simulink model "Lab03IntControleCOMPLETO"  (R2021a)
settings: Solver=ode45  StartTime=0.0  StopTime=150  RelTol=1e-3  EnableMultiTasking=on
settings Model: Creator=13199959938  LastModifiedBy=Usuario
settings SolverCC: AlgebraicLoopSolver=TrustRegion
settings DataIOCC: LimitDataPoints=on  SaveFormat=Array  ReturnWorkspaceOutputs=off
settings OptimizationCC: LifeSpan=inf
settings DebuggingCC: UnderspecifiedInitializationDetection=Classic  MergeDetectMultiDrivingBlocksExec=none  SolverPrmCheckMsg=warning  StateNameClashWarn=warning  SFUnexpectedBacktrackingDiag=warning  SFNoUnconditionalDefaultTransitionDiag=warning  SFExecutionAtInitializationDiag=none  SFMachineParentedDataDiag=warning  ArithmeticOperatorsInVariantConditions=warning
settings HardwareCC: ProdBitPerPointer=32  ProdBitPerSizeT=32  ProdBitPerPtrDiffT=32  ProdLargestAtomicFloat=None  ProdIntDivRoundTo=Undefined  ProdEndianess=Unspecified  ProdWordSize=32  ProdHWDeviceType=32-bit Generic
settings ModelReferenceCC: PropagateSignalLabelsOutOfModel=off
settings SFSimCC: SimUseLocalCustomCode=off  CustomCodeUndefinedFunction=UseInterfaceOnly
settings RTWCC: RTWUseLocalCustomCode=off
settings CodeAppCC: StateflowObjectComments=on
settings GRTTargetCC: TargetLangStandard=C89/C90 (ANSI)
settings ConfigComp: CovMetricSettings=dw  CovSaveCumulativeToWorkspaceVar=on  CovSaveSingleToWorkspaceVar=on  CovExternalEMLEnable=off

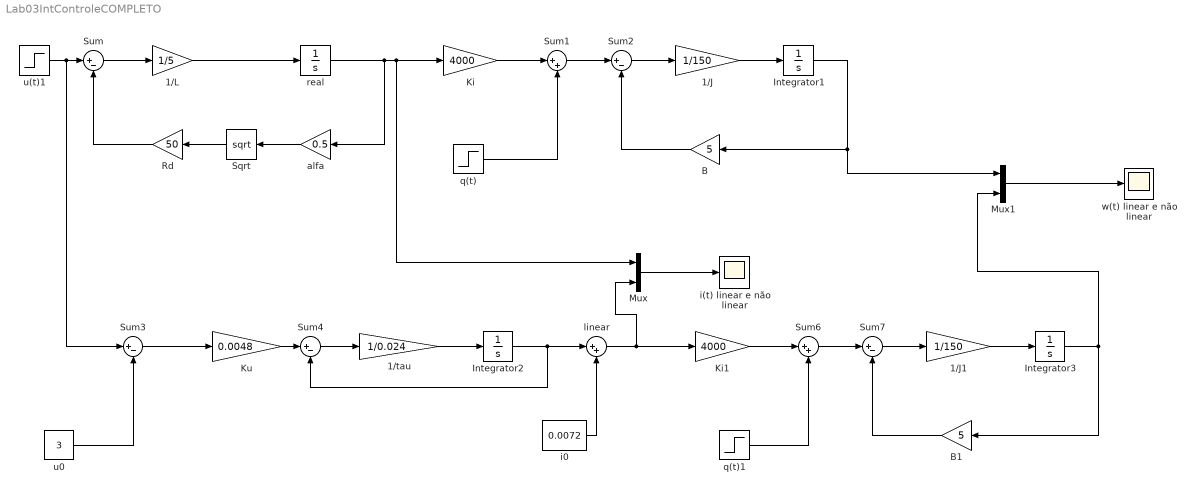
== system Lab03IntControleCOMPLETO ==
  1/J : Gain  Gain=1/150
  1/J1 : Gain  Gain=1/150
  1/L : Gain  Gain=1/5
  1/tau : Gain  Gain=1/0.024
  B : Gain  Gain=5
  B1 : Gain  Gain=5
  Integrator1 : Integrator
  Integrator2 : Integrator
  Integrator3 : Integrator
  Ki : Gain  Gain=4000
  Ki1 : Gain  Gain=4000
  Ku : Gain  Gain=0.0048
  Mux : Mux  Inputs=2
  Mux1 : Mux  Inputs=2
  Rd : Gain  Gain=50
  Sqrt : Sqrt  SaturateOnIntegerOverflow=on
  Sum{,2..4,7} (5 alike) : Sum  Inputs=|+-
  Sum1 : Sum  Inputs=|++
  Sum6 : Sum  Inputs=|++
  alfa : Gain  Gain=0.5
  i(t) linear e não linear : Scope
  i0 : Constant  Value=0.0072
  linear : Sum  Inputs=|++
  q(t) : Step  Time=50  After=0  SampleTime=0
  q(t)1 : Step  Time=50  SampleTime=0
  real : Integrator
  u(t)1 : Step  Time=50  Before=3  After=4.5  SampleTime=0
  u0 : Constant  Value=3
  w(t) linear e não linear : Scope
  wires:
  Rd/1 -> Sum/2
  Sum/1 -> 1/L/1
  1/L/1 -> real/1
  Sqrt/1 -> Rd/1
  alfa/1 -> Sqrt/1
  real/1 -> alfa/1, Mux/1, Ki/1
  Ki/1 -> Sum1/1
  Sum1/1 -> Sum2/1
  Sum2/1 -> 1/J/1
  1/J/1 -> Integrator1/1
  B/1 -> Sum2/2
  Integrator1/1 -> Mux1/1, B/1
  u0/1 -> Sum3/2
  Integrator2/1 -> Sum4/2, linear/1
  i0/1 -> linear/2
  Mux/1 -> i(t) linear e não linear/1
  Sum3/1 -> Ku/1
  Ku/1 -> Sum4/1
  Sum4/1 -> 1/tau/1
  1/tau/1 -> Integrator2/1
  q(t)1/1 -> Sum6/2
  Ki1/1 -> Sum6/1
  Sum6/1 -> Sum7/1
  Sum7/1 -> 1/J1/1
  1/J1/1 -> Integrator3/1
  B1/1 -> Sum7/2
  Integrator3/1 -> B1/1, Mux1/2
  Mux1/1 -> w(t) linear e não linear/1
  q(t)/1 -> Sum1/2
  linear/1 -> Mux/2, Ki1/1
  u(t)1/1 -> Sum3/1, Sum/1
